simulink model "sm_motor_grader_Drive_Steer"  (R2024b)
settings: Solver=daessc  StartTime=0.0  StopTime=stopTime  RelTol=1e-3  AbsTol=1e-3  EnableMultiTasking=on
PostLoadFcn:
  | [activeTestCmds,motGradParams,stopTime] = sm_motor_grader_define_test(motGradParams,'GradingTest');
StartFcn:
  | tic
StopFcn:
  | Elapsed_Sim_Time = toc;
undefined symbols (not defined in the file): Art, LnL, LnR, motGradParams, RFL, RFR, RRL, RRR, StrL, StrR
libraries: sm_motor_grader_lib x18, sm_lib x11, nesl_utility x8, fl_lib x2, sm_vehicle_utilities_lib x2
(part 1 of 2)
settings Model: Creator=smiller  LastModifiedBy=smiller
settings SolverCC: AutoScaleAbsTol=off  MaxConsecutiveMinStep=5  AlgebraicLoopSolver=TrustRegion  MaxZcPerStep=1
settings DataIOCC: LimitDataPoints=on  MaxDataPoints=10000  ReturnWorkspaceOutputs=off  SignalLoggingName=logsout_sm_motor_grader_Drive_Steer
settings OptimizationCC: ReuseModelBlockBuffer=off  LifeSpan=inf
settings DebuggingCC: UnconnectedInputMsg=warning  UnconnectedOutputMsg=warning  UnconnectedLineMsg=warning  AllowSymbolicDim=off  SubsystemReferenceDiagnosticForUnitTest=warning  SFUnexpectedBacktrackingDiag=warning  SFNoUnconditionalDefaultTransitionDiag=warning  SFExecutionAtInitializationDiag=none  ArithmeticOperatorsInVariantConditions=warning
settings ModelReferenceCC: EnableRefExpFcnMdlSchedulingChecks=on
settings SFSimCC: SimUseLocalCustomCode=off  CustomCodeUndefinedFunction=UseInterfaceOnly
settings RTWCC: RTWUseLocalCustomCode=off  GPUComputeCapability=3.5  DLArmComputeVersion=19.05
settings CodeAppCC: StateflowObjectComments=on
settings GRTTargetCC: TargetLangStandard=C89/C90 (ANSI)
settings ConfigComp: CovMetricSettings=dw  CovSaveCumulativeToWorkspaceVar=on  CovSaveSingleToWorkspaceVar=on  CovExternalEMLEnable=off  CovSFcnEnable=off
settings SimscapeCC: SimscapeLogType=all  SimscapeLogSimulationStatistics=on  SimscapeLogName=simlog_sm_motor_grader_Drive_Steer  SimscapeLogLimitData=off  SimscapeLogDataHistory=10000
settings DiagnosticsConfigSet: SimMechanicsConflictingReferenceFrames=none
settings ExplorerConfigSet: InternalSimMechanicsExplorerSettings="<ExplorerConfiguration><canonicalview>default</canonicalview><AnimationSetting><BasePlaybackSpeed>1.0</BasePlaybackSpeed><PlaybackSpeedFactor>2.0</PlaybackSpeedFactor></AnimationSetting><TilePanel><TileInfo><Tiles Columns=\"2\" Count=\"3\" Rows=\"2\"><Column Weight=\"0.5281\"/><Column Weight=\"0.4719\"/><Row Weight=\"0.5\"/><Row Weight=\"0.5\"/><Tile Height=\"1\" Width=\"1\" X=\"0\" Y=\"0\"/><Tile Height=\"1\" Width=\"1\" X=\"0\" Y=\"1\"/><Tile Height=\"2\" Width=\"1\" X=\"1\" Y=\"0\"/></Tiles></TileInfo><SceneInfo><SceneViewer><BGColor><R>1</R><G>1</G><B>1</B></BGColor><Camera><DoPerspective>on</DoPerspective><Position><X>185.119059192113696</X><Y>-6.61432654410976184</Y><Z>13.0658786835999603</Z></Position><Center><X>185.119059192113696</X><Y>-6.61432654410976184</Y><Z>12.0658786835999603</Z></Center><Up><X>0</X><Y>1</Y><Z>0</Z></Up><ViewLimDist>1</ViewLimDist><YLim>0.466307658154998583</YLim><XLim>1.09358272855567273</XLim></Camera></SceneViewer><SceneViewer><BGColor><R>1</R><G>1</G><B>1</B></BGColor><Camera><DoPerspective>on</DoPerspective><Position><X>190.2390591921137</X><Y>-12.2143265441097615</Y><Z>2.79921201693329458</Z></Position><Center><X>189.581235564168225</X><Y>-11.4948319510444055</Y><Z>2.57651130955592267</Z></Center><Up><X>-0.15027157805512012</X><Y>0.164359538497787616</Y><Z>0.974886862632591944</Z></Up><ViewLimDist>1</ViewLimDist><YLim>0.466307658154998583</YLim><XLim>1.09358272855567273</XLim></Camera></SceneViewer><SceneViewer><BGColor><R>1</R><G>1</G><B>1</B></BGColor><Camera><DoPerspective>on</DoPerspective><Position><X>192.619059192113696</X><Y>-6.61432654410976006</Y><Z>2.66587868359996127</Z></Position><Center><X>191.641066355689389</X><Y>-6.61432654410976006</Y><Z>2.45724021182944252</Z></Center><Up><X>-0.208638471770518946</X><Y>-2.55508436632761321e-17</Y><Z>0.977992836424307566</Z></Up><ViewLimDist>1</ViewLimDist><YLim>0.466307658154998583</YLim><XLim>0.480190723283956511</XLim></Camera></SceneViewer></SceneInfo></TilePanel><MechEditorPanel><Cameras><Camera><Id>Camera1</Id><Value><Name>Track FixO FR</Name><NativeCamera><PositionTrackingFeature>Motor_Grader.Vehicle.Camera_Frames.Frame_FixO_FR.R</PositionTrackingFeature><CenterTrackingFeature>Motor_Grader.Vehicle.Camera_Frames.Frame_FixO_FR.R</CenterTrackingFeature><UpVectorTrackingFeature>Motor_Grader.Vehicle.Camera_Frames.Frame_FixO_FR.R</UpVectorTrackingFeature><CenterTrackingOrigin>off</CenterTrackingOrigin><CenterTrackingDirection>+X</CenterTrackingDirection><UpVectorTrackingDirection>+Z</UpVectorTrackingDirection></NativeCamera></Value></Camera><Camera><Id>Camera2</Id><Value><Name>Track FixO Right</Name><NativeCamera><PositionTrackingFeature>Motor_Grader.Vehicle.Camera_Frames.Frame_FixO_Right.R</PositionTrackingFeature><CenterTrackingFeature>Motor_Grader.Vehicle.Camera_Frames.Frame_FixO_Right.R</CenterTrackingFeature><UpVectorTrackingFeature>Motor_Grader.Vehicle.Camera_Frames.Frame_FixO_Right.R</UpVectorTrackingFeature><CenterTrackingOrigin>off</CenterTrackingOrigin><CenterTrackingDirection>+X</CenterTrackingDirection><UpVectorTrackingDirection>+Z</UpVectorTrackingDirection></NativeCamera></Value></Camera><Camera><Id>Camera3</Id><Value><Name>Track FixO RR</Name><NativeCamera><PositionTrackingFeature>Motor_Grader.Vehicle.Camera_Frames.Frame_FixO_RR.R</PositionTrackingFeature><CenterTrackingFeature>Motor_Grader.Vehicle.Camera_Frames.Frame_FixO_RR.R</CenterTrackingFeature><UpVectorTrackingFeature>Motor_Grader.Vehicle.Camera_Frames.Frame_FixO_RR.R</UpVectorTrackingFeature><CenterTrackingOrigin>off</CenterTrackingOrigin><CenterTrackingDirection>+X</CenterTrackingDirection><UpVectorTrackingDirection>+Z</UpVectorTrackingDirection></NativeCamera></Value></Camera><Camera><Id>Camera4</Id><Value><Name>Track FixO RL</Name><NativeCamera><PositionTrackingFeature>Motor_Grader.Vehicle.Camera_Frames.Frame_FixO_RL.R</PositionTrackingFeature><CenterTrackingFeature>Motor_Grader.Vehicle.Camera_Frames.Frame_FixO_RL.R</CenterTrackingFeature><UpVectorTrackingFeature>Motor_Grader.Vehicle.Camera_Frames.Frame_FixO_RL.R</UpVectorTrackingFeature><CenterTrackingOrigin>off</CenterTrackingOrigin><CenterTrackingDirection>+X</CenterTrackingDirection><UpVectorTrackingDirection>+Z</UpVectorTrackingDirection></NativeCamera></Value></Camera><Camera><Id>Camera5</Id><Value><Name>Track FixO Left</Name><NativeCamera><PositionTrackingFeature>Motor_Grader.Vehicle.Camera_Frames.Frame_FixO_Left.R</PositionTrackingFeature><CenterTrackingFeature>Motor_Grader.Vehicle.Camera_Frames.Frame_FixO_Left.R</CenterTrackingFeature><UpVectorTrackingFeature>Motor_Grader.Vehicle.Camera_Frames.Frame_FixO_Left.R</UpVectorTrackingFeature><CenterTrackingOrigin>off</CenterTrackingOrigin><CenterTrackingDirection>+X</CenterTrackingDirection><UpVectorTrackingDirection>+Z</UpVectorTrackingDirection></NativeCamera></Value></Camera><Camera><Id>Camera6</Id><Value><Name>Track FixO FL</Name><NativeCamera><PositionTrackingFeature>Motor_Grader.Vehicle.Camera_Frames.Frame_FixO_FL.R</PositionTrackingFeature><CenterTrackingFeature>Motor_Grader.Vehicle.Camera_Frames.Frame_FixO_FL.R</CenterTrackingFeature><UpVectorTrackingFeature>Motor_Grader.Vehicle.Camera_Frames.Frame_FixO_FL.R</UpVectorTrackingFeature><CenterTrackingOrigin>off</CenterTrackingOrigin><CenterTrackingDirection>+X</CenterTrackingDirection><UpVectorTrackingDirection>+Z</UpVectorTrackingDirection></NativeCamera></Value></Camera><Camera><Id>Camera7</Id><Value><Name>Track FixO Top</Name><NativeCamera><PositionTrackingFeature>Motor_Grader.Vehicle.Camera_Frames.Frame_FixO_Top.R</PositionTrackingFeature><CenterTrackingFeature>Motor_Grader.Vehicle.Camera_Frames.Frame_FixO_Top.R</CenterTrackingFeature><UpVectorTrackingFeature>Motor_Grader.Vehicle.Camera_Frames.Frame_FixO_Top.R</UpVectorTrackingFeature><CenterTrackingOrigin>off</CenterTrackingOrigin><CenterTrackingDirection>+X</CenterTrackingDirection><UpVectorTrackingDirection>+Z</UpVectorTrackingDirection></NativeCamera></Value></Camera><Camera><Id>Camera8</Id><Value><Name>Track FixO Front</Name><NativeCamera><PositionTrackingFeature>Motor_Grader.Vehicle.Camera_Frames.Frame_FixO_Front.R</PositionTrackingFeature><CenterTrackingFeature>Motor_Grader.Vehicle.Camera_Frames.Frame_FixO_Front.R</CenterTrackingFeature><UpVectorTrackingFeature>Motor_Grader.Vehicle.Camera_Frames.Frame_FixO_Front.R</UpVectorTrackingFeature><CenterTrackingOrigin>off</CenterTrackingOrigin><CenterTrackingDirection>+X</CenterTrackingDirection><UpVectorTrackingDirection>+Z</UpVectorTrackingDirection></NativeCamera></Value></Camera><Camera><Id>Camera9</Id><Value><Name>Track FixO Rear</Name><NativeCamera><PositionTrackingFeature>Motor_Grader.Vehicle.Camera_Frames.Frame_FixO_Rear.R</PositionTrackingFeature><CenterTrackingFeature>Motor_Grader.Vehicle.Camera_Frames.Frame_FixO_Rear.R</CenterTrackingFeature><UpVectorTrackingFeature>Motor_Grader.Vehicle.Camera_Frames.Frame_FixO_Rear.R</UpVectorTrackingFeature><CenterTrackingOrigin>off</CenterTrackingOrigin><CenterTrackingDirection>+X</CenterTrackingDirection><UpVectorTrackingDirection>+Z</UpVectorTrackingDirection></NativeCamera></Value></Camera><Camera><Id>Camera10</Id><Value><Name>Track FR</Name><NativeCamera><PositionTrackingFeature>Motor_Grader.Vehicle.Camera_Frames.Frame_FR.R</PositionTrackingFeature><CenterTrackingFeature>Motor_Grader.Vehicle.Camera_Frames.Frame_FR.R</CenterTrackingFeature><UpVectorTrackingFeature>Motor_Grader.Vehicle.Camera_Frames.Frame_FR.R</UpVectorTrackingFeature><CenterTrackingOrigin>off</CenterTrackingOrigin><CenterTrackingDirection>+X</CenterTrackingDirection><UpVectorTrackingDirection>+Z</UpVectorTrackingDirection></NativeCamera></Value></Camera><Camera><Id>Camera11</Id><Value><Name>Track Right</Name><NativeCamera><PositionTrackingFeature>Motor_Grader.Vehicle.Camera_Frames.Frame_Right.R</PositionTrackingFeature><CenterTrackingFeature>Motor_Grader.Vehicle.Camera_Frames.Frame_Right.R</CenterTrackingFeature><UpVectorTrackingFeature>Motor_Grader.Vehicle.Camera_Frames.Frame_Right.R</UpVectorTrackingFeature><CenterTrackingOrigin>off</CenterTrackingOrigin><CenterTrackingDirection>+X</CenterTrackingDirection><UpVectorTrackingDirection>+Z</UpVectorTrackingDirection></NativeCamera></Value></Camera><Camera><Id>Camera12</Id><Value><Name>Track RR</Name><NativeCamera><PositionTrackingFeature>Motor_Grader.Vehicle.Camera_Frames.Frame_RR.R</PositionTrackingFeature><CenterTrackingFeature>Motor_Grader.Vehicle.Camera_Frames.Frame_RR.R</CenterTrackingFeature><UpVectorTrackingFeature>Motor_Grader.Vehicle.Camera_Frames.Frame_RR.R</UpVectorTrackingFeature><CenterTrackingOrigin>off</CenterTrackingOrigin><CenterTrackingDirection>+X</CenterTrackingDirection><UpVectorTrackingDirection>+Z</UpVectorTrackingDirection></NativeCamera></Value></Camera><Camera><Id>Camera13</Id><Value><Name>Track RL</Name><NativeCamera><PositionTrackingFeature>Motor_Grader.Vehicle.Camera_Frames.Frame_RL.R</PositionTrackingFeature><CenterTrackingFeature>Motor_Grader.Vehicle.Camera_Frames.Frame_RL.R</CenterTrackingFeature><UpVectorTrackingFeature>Motor_Grader.Vehicle.Camera_Frames.Frame_RL.R</UpVectorTrackingFeature><CenterTrackingOrigin>off</CenterTrackingOrigin><CenterTrackingDirection>+X</CenterTrackingDirection><UpVectorTrackingDirection>+Z</UpVectorTrackingDirection></NativeCamera></Value></Camera><Camera><Id>Camera14</Id><Value><Name>Track Left</Name><NativeCamera><PositionTrackingFeature>Motor_Grader.Vehicle.Camera_Frames.Frame_Left.R</PositionTrackingFeature><CenterTrackingFeature>Motor_Grader.Vehicle.Camera_Frames.Frame_Left.R</CenterTrackingFeature><UpVectorTrackingFeature>Motor_Grader.Vehicle.Camera_Frames.Frame_Left.R</UpVectorTrackingFeature><CenterTrackingOrigin>off</CenterTrackingOrigin><CenterTrackingDirection>+X</CenterTrackingDirection><UpVectorTrackingDirection>+Z</UpVectorTrackingDirection></NativeCamera></Value></Camera><Camera><Id>Camera15</Id><Value><Name>Track FL</Name><NativeCamera><PositionTrackingFeature>Motor_Grader.Vehicle.Camera_Frames.Frame_FL.R</PositionTrackingFeature><CenterTrackingFeature>Motor_Grader.Vehicle.Camera_Frames.Frame_FL.R</CenterTrackingFeature><UpVectorTrackingFeature>Motor_Grader.Vehicle.Camera_Frames.Frame_FL.R</UpVectorTrackingFeature><CenterTrackingOrigin>off</CenterTrackingOrigin><CenterTrackingDirection>+X</CenterTrackingDirection><UpVectorTrackingDirection>+Z</UpVectorTrackingDirection></NativeCamera></Value></Camera><Camera><Id>Camera16</Id><Value><Name>Track Top</Name><NativeCamera><PositionTrackingFeature>Motor_Grader.Vehicle.Camera_Frames.Frame_Top.R</PositionTrackingFeature><CenterTrackingFeature>Motor_Grader.Vehicle.Camera_Frames.Frame_Top.R</CenterTrackingFeature><UpVectorTrackingFeature>Motor_Grader.Vehicle.Camera_Frames.Frame_Top.R</UpVectorTrackingFeature><CenterTrackingOrigin>off</CenterTrackingOrigin><CenterTrackingDirection>+X</CenterTrackingDirection><UpVectorTrackingDirection>+Z</UpVectorTrackingDirection></NativeCamera></Value></Camera><Camera><Id>Camera17</Id><Value><Name>Track Front</Name><NativeCamera><PositionTrackingFeature>Motor_Grader.Vehicle.Camera_Frames.Frame_Front.R</PositionTrackingFeature><CenterTrackingFeature>Motor_Grader.Vehicle.Camera_Frames.Frame_Front.R</CenterTrackingFeature><UpVectorTrackingFeature>Motor_Grader.Vehicle.Camera_Frames.Frame_Front.R</UpVectorTrackingFeature><CenterTrackingOrigin>off</CenterTrackingOrigin><CenterTrackingDirection>+X</CenterTrackingDirection><UpVectorTrackingDirection>+Z</UpVectorTrackingDirection></NativeCamera></Value></Camera><Camera><Id>Camera18</Id><Value><Name>Track Rear</Name><NativeCamera><PositionTrackingFeature>Motor_Grader.Vehicle.Camera_Frames.Frame_Rear.R</PositionTrackingFeature><CenterTrackingFeature>Motor_Grader.Vehicle.Camera_Frames.Frame_Rear.R</CenterTrackingFeature><UpVectorTrackingFeature>Motor_Grader.Vehicle.Camera_Frames.Frame_Rear.R</UpVectorTrackingFeature><CenterTrackingOrigin>off</CenterTrackingOrigin><CenterTrackingDirection>+X</CenterTrackingDirection><UpVectorTrackingDirection>+Z</UpVectorTrackingDirection></NativeCamera></Value></Camera><Camera><Id>Camera19</Id><Value><Name>Track Blade Front</Name><NativeCamera><PositionTrackingFeature>Motor_Grader.Vehicle.Camera_Frames.Frame_SuspF.R</PositionTrackingFeature><CenterTrackingFeature>Motor_Grader.Vehicle.Camera_Frames.Frame_SuspF.R</CenterTrackingFeature><UpVectorTrackingFeature>Motor_Grader.Vehicle.Camera_Frames.Frame_SuspF.R</UpVectorTrackingFeature><CenterTrackingOrigin>off</CenterTrackingOrigin><CenterTrackingDirection>+X</CenterTrackingDirection><UpVectorTrackingDirection>+Z</UpVectorTrackingDirection></NativeCamera></Value></Camera><Camera><Id>Camera20</Id><Value><Name>Track Blade Rear</Name><NativeCamera><PositionTrackingFeature>Motor_Grader.Vehicle.Camera_Frames.Frame_SuspR.R</PositionTrackingFeature><CenterTrackingFeature>Motor_Grader.Vehicle.Camera_Frames.Frame_SuspR.R</CenterTrackingFeature><UpVectorTrackingFeature>Motor_Grader.Vehicle.Camera_Frames.Frame_SuspR.R</UpVectorTrackingFeature><CenterTrackingOrigin>off</CenterTrackingOrigin><CenterTrackingDirection>+X</CenterTrackingDirection><UpVectorTrackingDirection>+Z</UpVectorTrackingDirection></NativeCamera></Value></Camera><Camera><Id>Camera21</Id><Value><Name>Track Wheel FR</Name><NativeCamera><PositionTrackingFeature>Motor_Grader.Vehicle.Camera_Frames.Frame_Wheel_FR.R</PositionTrackingFeature><CenterTrackingFeature>Motor_Grader.Vehicle.Camera_Frames.Frame_Wheel_FR.R</CenterTrackingFeature><UpVectorTrackingFeature>Motor_Grader.Vehicle.Camera_Frames.Frame_Wheel_FR.R</UpVectorTrackingFeature><CenterTrackingOrigin>off</CenterTrackingOrigin><CenterTrackingDirection>+X</CenterTrackingDirection><UpVectorTrackingDirection>+Z</UpVectorTrackingDirection></NativeCamera></Value></Camera><Camera><Id>Camera22</Id><Value><Name>Track Blade Right</Name><NativeCamera><PositionTrackingFeature>Motor_Grader.Vehicle.Camera_Frames.Frame_Wheel_RR.R</PositionTrackingFeature><CenterTrackingFeature>Motor_Grader.Vehicle.Camera_Frames.Frame_Wheel_RR.R</CenterTrackingFeature><UpVectorTrackingFeature>Motor_Grader.Vehicle.Camera_Frames.Frame_Wheel_RR.R</UpVectorTrackingFeature><CenterTrackingOrigin>off</CenterTrackingOrigin><CenterTrackingDirection>+X</CenterTrackingDirection><UpVectorTrackingDirection>+Z</UpVectorTrackingDirection></NativeCamera></Value></Camera><Camera><Id>Camera23</Id><Value><Name>Track Blade Left</Name><NativeCamera><PositionTrackingFeature>Motor_Grader.Vehicle.Camera_Frames.Frame_Wheel_RL.R</PositionTrackingFeature><CenterTrackingFeature>Motor_Grader.Vehicle.Camera_Frames.Frame_Wheel_RL.R</CenterTrackingFeature><UpVectorTrackingFeature>Motor_Grader.Vehicle.Camera_Frames.Frame_Wheel_RL.R</UpVectorTrackingFeature><CenterTrackingOrigin>off</CenterTrackingOrigin><CenterTrackingDirection>+X</CenterTrackingDirection><UpVectorTrackingDirection>+Z</UpVectorTrackingDirection></NativeCamera></Value></Camera><Camera><Id>Camera24</Id><Value><Name>Track Wheel FL</Name><NativeCamera><PositionTrackingFeature>Motor_Grader.Vehicle.Camera_Frames.Frame_Wheel_FL.R</PositionTrackingFeature><CenterTrackingFeature>Motor_Grader.Vehicle.Camera_Frames.Frame_Wheel_FL.R</CenterTrackingFeature><UpVectorTrackingFeature>Motor_Grader.Vehicle.Camera_Frames.Frame_Wheel_FL.R</UpVectorTrackingFeature><CenterTrackingOrigin>off</CenterTrackingOrigin><CenterTrackingDirection>+X</CenterTrackingDirection><UpVectorTrackingDirection>+Z</UpVectorTrackingDirection></NativeCamera></Value></Camera><Camera><Id>Camera25</Id><Value><Name>View Seat</Name><NativeCamera><PositionTrackingFeature>Motor_Grader.Vehicle.Camera_Frames.Frame_View_Seat_FL.R</PositionTrackingFeature><CenterTrackingFeature>Motor_Grader.Vehicle.Camera_Frames.Frame_View_Seat_FL.R</CenterTrackingFeature><UpVectorTrackingFeature>Motor_Grader.Vehicle.Camera_Frames.Frame_View_Seat_FL.R</UpVectorTrackingFeature><CenterTrackingOrigin>off</CenterTrackingOrigin><CenterTrackingDirection>+X</CenterTrackingDirection><UpVectorTrackingDirection>+Z</UpVectorTrackingDirection></NativeCamera></Value></Camera><Camera><Id>Camera26</Id><Value><Name>View Seat FR</Name><NativeCamera><PositionTrackingFeature>Motor_Grader.Vehicle.Camera_Frames.Frame_View_Seat_FR.R</PositionTrackingFeature><CenterTrackingFeature>Motor_Grader.Vehicle.Camera_Frames.Frame_View_Seat_FR.R</CenterTrackingFeature><UpVectorTrackingFeature>Motor_Grader.Vehicle.Camera_Frames.Frame_View_Seat_FR.R</UpVectorTrackingFeature><CenterTrackingOrigin>off</CenterTrackingOrigin><CenterTrackingDirection>+X</CenterTrackingDirection><UpVectorTrackingDirection>+Z</UpVectorTrackingDirection></NativeCamera></Value></Camera><Camera><Id>Camera27</Id><Value><Name>View Susp FR</Name><NativeCamera><PositionTrackingFeature>Motor_Grader.Vehicle.Camera_Frames.Frame_View_Susp_FR.R</PositionTrackingFeature><CenterTrackingFeature>Motor_Grader.Vehicle.Camera_Frames.Frame_View_Susp_FR.R</CenterTrackingFeature><UpVectorTrackingFeature>Motor_Grader.Vehicle.Camera_Frames.Frame_View_Susp_FR.R</UpVectorTrackingFeature><CenterTrackingOrigin>off</CenterTrackingOrigin><CenterTrackingDirection>+X</CenterTrackingDirection><UpVectorTrackingDirection>+Z</UpVectorTrackingDirection></NativeCamera></Value></Camera><Camera><Id>Camera28</Id><Value><Name>View SaddleR</Name><NativeCamera><PositionTrackingFeature>Motor_Grader.Vehicle.Camera_Frames.Frame_View_Susp_RR.R</PositionTrackingFeature><CenterTrackingFeature>Motor_Grader.Vehicle.Camera_Frames.Frame_View_Susp_RR.R</CenterTrackingFeature><UpVectorTrackingFeature>Motor_Grader.Vehicle.Camera_Frames.Frame_View_Susp_RR.R</UpVectorTrackingFeature><CenterTrackingOrigin>off</CenterTrackingOrigin><CenterTrackingDirection>+X</CenterTrackingDirection><UpVectorTrackingDirection>+Z</UpVectorTrackingDirection></NativeCamera></Value></Camera><Camera><Id>Camera29</Id><Value><Name>View SaddleL</Name><NativeCamera><PositionTrackingFeature>Motor_Grader.Vehicle.Camera_Frames.Frame_View_Susp_RL.R</PositionTrackingFeature><CenterTrackingFeature>Motor_Grader.Vehicle.Camera_Frames.Frame_View_Susp_RL.R</CenterTrackingFeature><UpVectorTrackingFeature>Motor_Grader.Vehicle.Camera_Frames.Frame_View_Susp_RL.R</UpVectorTrackingFeature><CenterTrackingOrigin>off</CenterTrackingOrigin><CenterTrackingDirection>+X</CenterTrackingDirection><UpVectorTrackingDirection>+Z</UpVectorTrackingDirection></NativeCamera></Value></Camera><Camera><Id>Camera30</Id><Value><Name>View Susp FL</Name><NativeCamera><PositionTrackingFeature>Motor_Grader.Vehicle.Camera_Frames.Frame_View_Susp_FL.R</PositionTrackingFeature><CenterTrackingFeature>Motor_Grader.Vehicle.Camera_Frames.Frame_View_Susp_FL.R</CenterTrackingFeature><UpVectorTrackingFeature>Motor_Grader.Vehicle.Camera_Frames.Frame_View_Susp_FL.R</UpVectorTrackingFeature><CenterTrackingOrigin>off</CenterTrackingOrigin><CenterTrackingDirection>+X</CenterTrackingDirection><UpVectorTrackingDirection>+Z</UpVectorTrackingDirection></NativeCamera></Value></Camera><Camera><Id>Camera31</Id><Value><Name>Dolly Camera</Name><NativeCamera><PositionTrackingFeature>Motor_Grader.Vehicle.Camera_Frames.Frame_Dolly.R</PositionTrackingFeature><CenterTrackingFeature>Motor_Grader.Vehicle.Camera_Frames.Frame_Dolly.R</CenterTrackingFeature><UpVectorTrackingFeature>Motor_Grader.Vehicle.Camera_Frames.Frame_Dolly.R</UpVectorTrackingFeature><CenterTrackingOrigin>off</CenterTrackingOrigin><CenterTrackingDirection>+X</CenterTrackingDirection><UpVectorTrackingDirection>+Z</UpVectorTrackingDirection></NativeCamera></Value></Camera><Camera><Id>Camera32</Id><Value><Name>Track Dolly Camera</Name><NativeCamera><PositionTrackingFeature>Motor_Grader.Vehicle.Camera_Frames.Frame_Dolly.R</PositionTrackingFeature><CenterTrackingFeature>Motor_Grader.Vehicle.Camera_Frames.Transform_Camera_Ref.F</CenterTrackingFeature><UpVectorTrackingFeature>Motor_Grader.Vehicle.Camera_Frames.World_Frame.W</UpVectorTrackingFeature><CenterTrackingOrigin>on</CenterTrackingOrigin><UpVectorTrackingDirection>+Z</UpVectorTrackingDirection></NativeCamera></Value></Camera></Cameras><GfxPanelCameraMap><MapElement CameraMLId=\"Camera7\" GfxPanelIndex=\"0\"/><MapElement CameraMLId=\"Camera1\" GfxPanelIndex=\"1\"/><MapElement CameraMLId=\"Camera8\" GfxPanelIndex=\"2\"/></GfxPanelCameraMap><VideoCreator><PlaybackSpeedRatio>1.0</PlaybackSpeedRatio><FrameRate>30</FrameRate><VideoFormat>MPEG-4</VideoFormat><FrameSize>[800 450]</FrameSize></VideoCreator></MechEditorPanel></ExplorerConfiguration>"

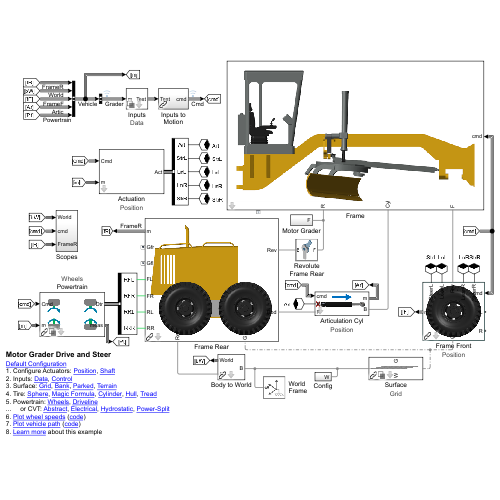
[thumbnail: Simulink's stored preview of the top-level diagram]
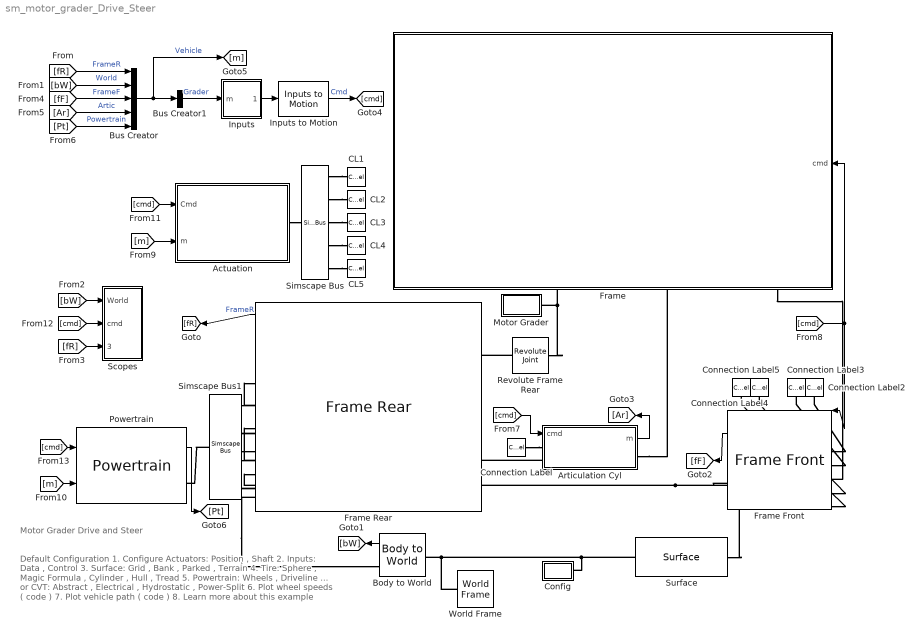
== system sm_motor_grader_Drive_Steer ==
  note: Motor Grader Drive and Steer
  note: Default Configuration
      | 1. Configure Actuators: Position , Shaft
      | 2. Inputs: Data , Control
      | 3. Surface: Grid , Bank , Parked , Terrain
      | 4. Tire: Sphere , Magic Formula , Cylinder , Hull , Tread
      | 5. Powertrain: Wheels , Driveline
      | ... or CVT: Abstract , Electrical , Hydrostatic , Power-Split
      | 6. Plot wheel speeds ( code )
      | 7. Plot vehicle path ( code )
      | 8. Learn more about this example
  Actuation : Subsystem  VariantControl=Actuation  mask{popup_actuator_model=Position}
      mask prompts: popup_actuator_model "Actuation Mode"
      mask init:
      | bh = gcb;
      | modestr = get_param(bh,'popup_actuator_model');
      | 
      | set_param([bh '/Actuator SteerL'],'LabelModeActiveChoice',modestr)
      | set_param([bh '/Actuator SteerR'],'LabelModeActiveChoice',modestr)
      | set_param([bh '/Actuator LeanL'],'LabelModeActiveChoice',modestr)
      | set_param([bh '/Actuator LeanR'],'LabelModeActiveChoice',modestr)
      settings: AttributesFormatString=%<popup_actuator_model>
      mask TypeOptions popup_actuator_model: Position | Shaft
  Articulation Cyl : Subsystem  mask{popup_actuator_model=Position}
      mask prompts: popup_actuator_model "Actuation Mode"
      mask init:
      | bh = gcb;
      | if(strcmp(get_param(bh,'popup_actuator_model'),'Shaft'))
      |     set_param([bh '/Actuator'],'LabelModeActiveChoice','Shaft')
      | else
      |     set_param([bh '/Actuator'],'LabelModeActiveChoice','Position')
      | end
      settings: AttributesFormatString=%<popup_actuator_model>
      mask TypeOptions popup_actuator_model: Position | Shaft
      mask Display:
      | bh = gcb;
      | if(strcmp(get_param(bh,'popup_actuator_model'),'Position'))
      |     image('sm_motor_grader_actuator_intfPosition_IMAGE.png')
      | else
      |     image('sm_motor_grader_actuator_intfShaft_IMAGE.png')
      | end
      | %image('sm_motor_grader_articCylRod_IMAGE.png')
  Body to World : sm_vehicle_utilities_lib/Body to World  Init=Init.Vehicle  SpecifyPosTarget=on
  Bus Creator : BusCreator  Inputs=5
  Bus Creator1 : BusCreator  Inputs=1
  CL1 : ConnectionLabel  Label=Art
  CL2 : ConnectionLabel  Label=StrL
  CL3 : ConnectionLabel  Label=LnL
  CL4 : ConnectionLabel  Label=LnR
  CL5 : ConnectionLabel  Label=StrR
  Config : Subsystem
  Connection Label : ConnectionLabel  Label=Art
  Connection Label2 : ConnectionLabel  Label=StrR
  Connection Label3 : ConnectionLabel  Label=LnR
  Connection Label4 : ConnectionLabel  Label=LnL
  Connection Label5 : ConnectionLabel  Label=StrL
  Frame : Subsystem
      settings: PortSchema="{\"entries\":[{\"content\":{\"sides\":[{\"content\":{},\"type\":\"ConnectorPlacement.EquallySpacedRectSide\",\"uuid\":\"956ff1aa-cf24-496e-9779-d98cb55dab7e\"},{\"content\":{\"connectorIds\":[\"RConn1\",\"RConn2\",\"RConn3\",\"RConn4\"],\"side\":\"RIGHT\"},\"type\":\"ConnectorPlacement.EquallySpacedRectSide\",\"uuid\":\"9c9b4268-8eee-41b9-b50a-4033054aa2f0\"},{\"content\":{\"side\":\"TOP\"},\"type\":\"ConnectorPlacement.EquallySpacedRectSide\",\"uuid\":\"ed4b7b74-ed0a-49ca-b139-bba335fa3413\"},{\"content\":{\"connectorIds\":[\"In1\"],\"side\":\"BOTTOM\"},\"type\":\"ConnectorPlacement.EquallySpacedRectSide\",\"uuid\":\"cd037d6e-8d6c-4a0e-a629-b4586db15f4a\"}]},\"type\":\"ConnectorPlacement.EquallySpacedConnector\",\"uuid\":\"3490148e-7dca-48b7-9597-0781f6c140f1\"}],\"packageUris\":[\"http://schema.mathworks.com/mf0/Connector/R2020b\"],\"version\":\"1.0\"}"
      mask Display: image('sm_motor_grader_frameCabBlade_IMAGE.png')
  Frame Front : sm_motor_grader_lib/Frame Front  popup_actuator_model=Position  popup_ground_contact=Magic Formula
      settings: AttributesFormatString=%<popup_actuator_model>
  Frame Rear : sm_motor_grader_lib/Frame Rear  popup_ground_contact=Magic Formula
  Inputs : Subsystem  Variant=on  VariantControlMode=label  VariantControl=Inputs  LabelModeActiveChoice=Data  mask{test_source=Data}
      mask prompts: test_source "Test Source"
      mask init:
      | bh = gcb;
      | data_source = get_param(bh,'test_source');
      | set_param(bh,'LabelModeActiveChoice',data_source)
      settings: AttributesFormatString=%<LabelModeActiveChoice>
      mask TypeOptions test_source: Data | Control
      mask Display: disp(' ')
  Inputs to Motion : sm_motor_grader_lib/Inputs to Motion  SystemSampleTime=-1  VariantActivationTime=update diagram  AllowFlexibleInterface=on  Latency=0  AutoFrameSizeCalculation=off
  Motor Grader : Subsystem
  Powertrain : sm_motor_grader_lib/Powertrain  VariantControl=Powertrain  LabelModeActiveChoice=Torque4  popup_powertrain_config=Wheels
      settings: AttributesFormatString=%<popup_powertrain_config>
  Revolute Frame Rear : sm_lib/Joints/Revolute Joint  JointMode=Normal  CompositeWrenchDir=FollowerOnBase  CompositeWrenchFrame=BaseFrame  SenseConstraintForce=off  SenseConstraintTorque=off  SenseTotalForce=off  SenseTotalTorque=off  PositionTargetSpecify=on  PositionTargetPriority=Low  PositionTargetValue=0  PositionTargetValueUnits=deg  VelocityTargetSpecify=off  VelocityTargetPriority=High  VelocityTargetValue=0  VelocityTargetValueUnits=deg/s  EquilibriumPosition=0  EquilibriumPositionUnits=deg  SpringStiffness=0  SpringStiffnessUnits=N*m/deg  DampingCoefficient=0  DampingCoefficientUnits=N*m/(deg/s)  LowerLimitSpecify=off  LowerLimitBound=-90  LowerLimitBoundUnits=deg  LowerLimitStiffness=1e4  LowerLimitStiffnessUnits=N*m/deg  LowerLimitDamping=10  LowerLimitDampingUnits=N*m/(deg/s)  LowerLimitTransitionRegionWidth=0.1  LowerLimitTransitionRegionWidthUnits=deg  UpperLimitSpecify=off  UpperLimitBound=90  UpperLimitBoundUnits=deg  UpperLimitStiffness=1e4  UpperLimitStiffnessUnits=N*m/deg  UpperLimitDamping=10  UpperLimitDampingUnits=N*m/(deg/s)  UpperLimitTransitionRegionWidth=0.1  UpperLimitTransitionRegionWidthUnits=deg  TorqueActuationMode=NoTorque  MotionActuationMode=ComputedMotion  SensePosition=off  SenseVelocity=off  SenseAcceleration=off  SenseTorqueForce=off  SenseLowerLimitTorqueForce=off  SenseUpperLimitTorqueForce=off
  Scopes : Subsystem
  Simscape Bus : SimscapeBus  HierarchyStrings=Art;StrL;LnL;LnR;StrR
  Simscape Bus1 : SimscapeBus  HierarchyStrings=RFL;RFR;RRL;RRR
  Surface : sm_motor_grader_lib/Surface  VariantControl=Grid  LabelModeActiveChoice=Grid  popup_surface_type=Grid
      settings: AttributesFormatString=%<popup_surface_type>
  World Frame : sm_lib/Frames and Transforms/World Frame
  wires:
  Frame Rear/1 -> [fR]  "FrameR"
  Bus Creator1/1 -> Inputs/1(m)  "Grader"
  Inputs to Motion/1 -> [cmd]  "Cmd"
  [fR] -> Bus Creator/1  "FrameR"
  Body to World/1 -> [bW]
  [bW] -> Bus Creator/2  "World"
  Articulation Cyl/1(m) -> [Ar]
  Frame Front/1 -> [fF]
  Inputs/1(Test) -> Inputs to Motion/1
  [fF] -> Bus Creator/3  "FrameF"
  [Ar] -> Bus Creator/4  "Artic"
  [cmd] -> Frame Front/1, Frame/1(cmd)
  [cmd] -> Articulation Cyl/1(cmd)
  [m] -> Actuation/2(m)
  [m] -> Powertrain/2
  [cmd] -> Actuation/1(Cmd)
  [cmd] -> Powertrain/1
  [bW] -> Scopes/1(World)
  [cmd] -> Scopes/2(cmd)
  [fR] -> Scopes/3(FrameR)
  Bus Creator/1 -> [m], Bus Creator1/1  "Vehicle"
  Powertrain/1 -> [Pt]
  [Pt] -> Bus Creator/5  "Powertrain"
  connections:
  Simscape Bus1/RConn1 -- Powertrain/RConn1
  Revolute Frame Rear/LConn1 -- Frame Rear/LConn1
  World Frame/RConn1 -- Surface/LConn1 -- Config/LConn1 -- Body to World/LConn1
  Frame Rear/RConn8 -- Body to World/RConn1
  Frame Front/RConn1 -- Surface/RConn1 -- Frame Rear/RConn7
  Frame Front/LConn6 -- Connection Label4/LConn1
  Frame Front/LConn3 -- Connection Label2/LConn1
  Frame Front/LConn7 -- Connection Label5/LConn1
  Frame Front/LConn4 -- Connection Label3/LConn1
  Revolute Frame Rear/RConn1 -- Frame/RConn2 -- Motor Grader/RConn1
  Articulation Cyl/LConn2 -- Frame Rear/LConn2
  Articulation Cyl/RConn1 -- Frame/RConn3
  Simscape Bus1/LConn1 -- Frame Rear/RConn3
  Simscape Bus1/LConn2 -- Frame Rear/RConn4
  Simscape Bus1/LConn3 -- Frame Rear/RConn5
  Simscape Bus1/LConn4 -- Frame Rear/RConn6
  Actuation/RConn1 -- Simscape Bus/RConn1
  Simscape Bus/LConn4 -- CL4/LConn1
  Simscape Bus/LConn5 -- CL5/LConn1
  Simscape Bus/LConn2 -- CL2/LConn1
  Simscape Bus/LConn1 -- CL1/LConn1
  Simscape Bus/LConn3 -- CL3/LConn1
  Connection Label/LConn1 -- Articulation Cyl/LConn1
  Frame/RConn4 -- Frame Front/LConn5

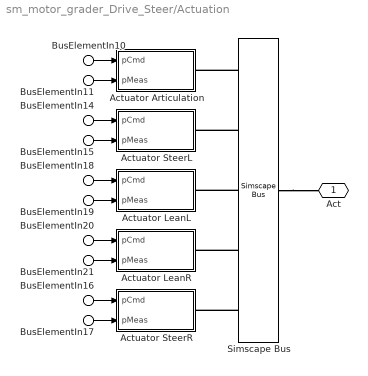
== system sm_motor_grader_Drive_Steer/Actuation ==
  BusElementIn10 : Inport  PortName=Cmd  Element=pArtic
  BusElementIn14 : Inport  PortName=Cmd  Element=pSteerL
  BusElementIn16 : Inport  PortName=Cmd  Element=pSteerR
  BusElementIn18 : Inport  PortName=Cmd  Element=pLeanL
  BusElementIn20 : Inport  PortName=Cmd  Element=pLeanR
  BusElementIn11 : Inport  Port=2  PortName=m  Element=Artic.p
  BusElementIn15 : Inport  Port=2  PortName=m  Element=FrameF.SteerL.p
  BusElementIn19 : Inport  Port=2  PortName=m  Element=FrameF.LeanL.p
  BusElementIn21 : Inport  Port=2  PortName=m  Element=FrameF.LeanR.p
  BusElementIn17 : Inport  Port=2  PortName=m  Element=FrameF.SteerR.p
  Actuator Articulation : Subsystem  Variant=on  VariantControlMode=label  VariantControl=Actuator Articulation  LabelModeActiveChoice=Position
  Actuator LeanL : Subsystem  Variant=on  VariantControlMode=label  VariantControl=Actuator LeanL  LabelModeActiveChoice=Position
  Actuator LeanR : Subsystem  Variant=on  VariantControlMode=label  VariantControl=Actuator LeanR  LabelModeActiveChoice=Position
  Actuator SteerL : Subsystem  Variant=on  VariantControlMode=label  VariantControl=Actuator SteerL  LabelModeActiveChoice=Position
  Actuator SteerR : Subsystem  Variant=on  VariantControlMode=label  VariantControl=Actuator SteerR  LabelModeActiveChoice=Position
  Simscape Bus : SimscapeBus  HierarchyStrings=Art;StrL;LnL;LnR;StrR
  Act : PMIOPort  Side=Right
  wires:
  BusElementIn21/1 -> Actuator LeanR/2(pMeas)
  BusElementIn20/1 -> Actuator LeanR/1(pCmd)
  BusElementIn19/1 -> Actuator LeanL/2(pMeas)
  BusElementIn18/1 -> Actuator LeanL/1(pCmd)
  BusElementIn17/1 -> Actuator SteerR/2(pMeas)
  BusElementIn16/1 -> Actuator SteerR/1(pCmd)
  BusElementIn15/1 -> Actuator SteerL/2(pMeas)
  BusElementIn14/1 -> Actuator SteerL/1(pCmd)
  BusElementIn11/1 -> Actuator Articulation/2(pMeas)
  BusElementIn10/1 -> Actuator Articulation/1(pCmd)
  connections:
  Simscape Bus/LConn4 -- Actuator LeanR/RConn1
  Simscape Bus/LConn3 -- Actuator LeanL/RConn1
  Simscape Bus/LConn5 -- Actuator SteerR/RConn1
  Simscape Bus/LConn2 -- Actuator SteerL/RConn1
  Simscape Bus/LConn1 -- Actuator Articulation/RConn1
  Simscape Bus/RConn1 -- Act/RConn1

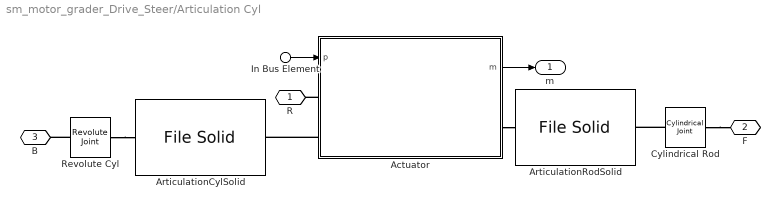
== system sm_motor_grader_Drive_Steer/Articulation Cyl ==
  In Bus Element : Inport  PortName=cmd  Element=pArtic
  Actuator : Subsystem  Variant=on  VariantControlMode=label  VariantControl=Position  LabelModeActiveChoice=Position
  ArticulationCylSolid : sm_lib/Body Elements/File Solid  ExtGeomFileName=ArticulationCylinder.step  UnitType=FromFile  ExtGeomFileUnits=m  StepReaderType=HEX  ExportConvexHullGeometry=off  InertiaType=CalculateFromGeometry  BasedOnType=Mass  Density=1000  DensityUnits=kg/m^3  Mass=motGradParams.articulation.cyl.mass  MassUnits=kg  CenterOfMass=[0 0 0]  CenterOfMassUnits=m  MomentsOfInertia=[1 1 1]  MomentsOfInertiaUnits=kg*m^2  ProductsOfInertia=[0 0 0]  ProductsOfInertiaUnits=kg*m^2  GraphicType=FromGeometry  MarkerShape=Sphere  MarkerSize=10  GraphicVisPropType=SimpleVisualProperties  GraphicDiffuseColor=mtrgrd.clr.artic_cyl  GraphicOpacity=0.5  GraphicSpecularColor=[0.5 0.5 0.5 1.0]  GraphicAmbientColor=[0.15 0.15 0.15 1.0]  GraphicEmissiveColor=[0.0 0.0 0.0 1.0]  GraphicShininess=75  DoExposeReferenceFrame=off  SerializedFrames=<Frames><Frame><Id>Frame1</Id><Value><Name>MainFrameRev</Name><Origin><Source>GeometricFeature</Source><FeatureName>circular curve 11</FeatureName></Origin><PrimaryAxis><DefinedDirection>-Z</DefinedDirection><Source>GeometricFeature</Source><SourceDirection>+Z</SourceDirection><FeatureName>segment 13</FeatureName></PrimaryAxis><SecondaryAxis><DefinedDirection>+X</DefinedDirection><Source>ReferenceFrame</Source><SourceDirection>+X</SourceDirection><FeatureName></FeatureName></SecondaryAxis></Value></Frame><Frame><Id>Frame2</Id><Value><Name>ArticulationCyl</Name><Origin><Source>GeometricFeature</Source><FeatureName>circular curve 5</FeatureName></Origin><PrimaryAxis><DefinedDirection>-Z</DefinedDirection><Source>GeometricFeature</Source><SourceDirection>+Z</SourceDirection><FeatureName>segment 7</FeatureName></PrimaryAxis><SecondaryAxis><DefinedDirection>+X</DefinedDirection><Source>ReferenceFrame</Source><SourceDirection>+X</SourceDirection><FeatureName></FeatureName></SecondaryAxis></Value></Frame></Frames>
  ArticulationRodSolid : sm_lib/Body Elements/File Solid  ExtGeomFileName=ArticulationPiston.step  UnitType=FromFile  ExtGeomFileUnits=m  StepReaderType=HEX  ExportConvexHullGeometry=off  InertiaType=CalculateFromGeometry  BasedOnType=Mass  Density=1000  DensityUnits=kg/m^3  Mass=motGradParams.articulation.rod.mass  MassUnits=kg  CenterOfMass=[0 0 0]  CenterOfMassUnits=m  MomentsOfInertia=[1 1 1]  MomentsOfInertiaUnits=kg*m^2  ProductsOfInertia=[0 0 0]  ProductsOfInertiaUnits=kg*m^2  GraphicType=FromGeometry  MarkerShape=Sphere  MarkerSize=10  GraphicVisPropType=SimpleVisualProperties  GraphicDiffuseColor=mtrgrd.clr.artic_rod  GraphicOpacity=1  GraphicSpecularColor=[0.5 0.5 0.5 1.0]  GraphicAmbientColor=[0.15 0.15 0.15 1.0]  GraphicEmissiveColor=[0.0 0.0 0.0 1.0]  GraphicShininess=75  DoExposeReferenceFrame=off  SerializedFrames=<Frames><Frame><Id>Frame1</Id><Value><Name>RearFrame</Name><Origin><Source>GeometricFeature</Source><FeatureName>circular curve 4</FeatureName></Origin><PrimaryAxis><DefinedDirection>+Z</DefinedDirection><Source>ReferenceFrame</Source><SourceDirection>+Z</SourceDirection><FeatureName></FeatureName></PrimaryAxis><SecondaryAxis><DefinedDirection>+X</DefinedDirection><Source>ReferenceFrame</Source><SourceDirection>+X</SourceDirection><FeatureName></FeatureName></SecondaryAxis></Value></Frame><Frame><Id>Frame2</Id><Value><Name>ArticulationCyl</Name><Origin><Source>GeometricFeature</Source><FeatureName>planar surface 1</FeatureName></Origin><PrimaryAxis><DefinedDirection>-Z</DefinedDirection><Source>GeometricFeature</Source><SourceDirection>+Z</SourceDirection><FeatureName>segment 10</FeatureName></PrimaryAxis><SecondaryAxis><DefinedDirection>+X</DefinedDirection><Source>ReferenceFrame</Source><SourceDirection>+X</SourceDirection><FeatureName></FeatureName></SecondaryAxis></Value></Frame></Frames>
  Cylindrical Rod : sm_lib/Joints/Cylindrical Joint  JointMode=Normal  CompositeWrenchDir=FollowerOnBase  CompositeWrenchFrame=BaseFrame  SenseConstraintForce=off  SenseConstraintTorque=off  SenseTotalForce=off  SenseTotalTorque=off  RzPositionTargetSpecify=off  RzPositionTargetPriority=High  RzPositionTargetValue=0  RzPositionTargetValueUnits=deg  RzVelocityTargetSpecify=off  RzVelocityTargetPriority=High  RzVelocityTargetValue=0  RzVelocityTargetValueUnits=deg/s  RzEquilibriumPosition=0  RzEquilibriumPositionUnits=deg  RzSpringStiffness=0  RzSpringStiffnessUnits=N*m/deg  RzDampingCoefficient=0  RzDampingCoefficientUnits=N*m/(deg/s)  RzLowerLimitSpecify=off  RzLowerLimitBound=-90  RzLowerLimitBoundUnits=deg  RzLowerLimitStiffness=1e4  RzLowerLimitStiffnessUnits=N*m/deg  RzLowerLimitDamping=10  RzLowerLimitDampingUnits=N*m/(deg/s)  RzLowerLimitTransitionRegionWidth=0.1  RzLowerLimitTransitionRegionWidthUnits=deg  RzUpperLimitSpecify=off  RzUpperLimitBound=90  RzUpperLimitBoundUnits=deg  RzUpperLimitStiffness=1e4  RzUpperLimitStiffnessUnits=N*m/deg  RzUpperLimitDamping=10  RzUpperLimitDampingUnits=N*m/(deg/s)  RzUpperLimitTransitionRegionWidth=0.1  RzUpperLimitTransitionRegionWidthUnits=deg  RzTorqueActuationMode=NoTorque  RzMotionActuationMode=ComputedMotion  RzSensePosition=off  RzSenseVelocity=off  RzSenseAcceleration=off  RzSenseTorqueForce=off  RzSenseLowerLimitTorqueForce=off  RzSenseUpperLimitTorqueForce=off  PzPositionTargetSpecify=off  PzPositionTargetPriority=High  PzPositionTargetValue=0  PzPositionTargetValueUnits=m  PzVelocityTargetSpecify=off  PzVelocityTargetPriority=High  PzVelocityTargetValue=0  PzVelocityTargetValueUnits=m/s  PzEquilibriumPosition=0  PzEquilibriumPositionUnits=m  PzSpringStiffness=0  PzSpringStiffnessUnits=N/m  PzDampingCoefficient=0  PzDampingCoefficientUnits=N/(m/s)  PzLowerLimitSpecify=off  PzLowerLimitBound=-1  PzLowerLimitBoundUnits=m  PzLowerLimitStiffness=1e6  PzLowerLimitStiffnessUnits=N/m  PzLowerLimitDamping=1e3  PzLowerLimitDampingUnits=N/(m/s)  PzLowerLimitTransitionRegionWidth=1e-4  PzLowerLimitTransitionRegionWidthUnits=m  PzUpperLimitSpecify=off  PzUpperLimitBound=1  PzUpperLimitBoundUnits=m  PzUpperLimitStiffness=1e6  PzUpperLimitStiffnessUnits=N/m  PzUpperLimitDamping=1e3  PzUpperLimitDampingUnits=N/(m/s)  PzUpperLimitTransitionRegionWidth=1e-4  PzUpperLimitTransitionRegionWidthUnits=m  PzTorqueActuationMode=NoTorque  PzMotionActuationMode=ComputedMotion  PzSensePosition=off  PzSenseVelocity=off  PzSenseAcceleration=off  PzSenseTorqueForce=off  PzSenseLowerLimitTorqueForce=off  PzSenseUpperLimitTorqueForce=off
  Revolute Cyl : sm_lib/Joints/Revolute Joint  JointMode=Normal  CompositeWrenchDir=FollowerOnBase  CompositeWrenchFrame=BaseFrame  SenseConstraintForce=off  SenseConstraintTorque=off  SenseTotalForce=off  SenseTotalTorque=off  PositionTargetSpecify=off  PositionTargetPriority=High  PositionTargetValue=0  PositionTargetValueUnits=deg  VelocityTargetSpecify=off  VelocityTargetPriority=High  VelocityTargetValue=0  VelocityTargetValueUnits=deg/s  EquilibriumPosition=0  EquilibriumPositionUnits=deg  SpringStiffness=0  SpringStiffnessUnits=N*m/deg  DampingCoefficient=0  DampingCoefficientUnits=N*m/(deg/s)  LowerLimitSpecify=off  LowerLimitBound=-90  LowerLimitBoundUnits=deg  LowerLimitStiffness=1e4  LowerLimitStiffnessUnits=N*m/deg  LowerLimitDamping=10  LowerLimitDampingUnits=N*m/(deg/s)  LowerLimitTransitionRegionWidth=0.1  LowerLimitTransitionRegionWidthUnits=deg  UpperLimitSpecify=off  UpperLimitBound=90  UpperLimitBoundUnits=deg  UpperLimitStiffness=1e4  UpperLimitStiffnessUnits=N*m/deg  UpperLimitDamping=10  UpperLimitDampingUnits=N*m/(deg/s)  UpperLimitTransitionRegionWidth=0.1  UpperLimitTransitionRegionWidthUnits=deg  TorqueActuationMode=NoTorque  MotionActuationMode=ComputedMotion  SensePosition=off  SenseVelocity=off  SenseAcceleration=off  SenseTorqueForce=off  SenseLowerLimitTorqueForce=off  SenseUpperLimitTorqueForce=off
  R : PMIOPort  Side=Left
  F : PMIOPort  Port=2  Side=Left
  B : PMIOPort  Port=3  Side=Right
  m : Outport
  wires:
  In Bus Element/1 -> Actuator/1(p)
  Actuator/1(m) -> m/1
  connections:
  Revolute Cyl/RConn1 -- ArticulationCylSolid/LConn1
  Revolute Cyl/LConn1 -- B/RConn1
  Cylindrical Rod/LConn1 -- F/RConn1
  Cylindrical Rod/RConn1 -- ArticulationRodSolid/LConn1
  Actuator/LConn1 -- R/RConn1
  Actuator/LConn2 -- ArticulationCylSolid/RConn1
  Actuator/RConn1 -- ArticulationRodSolid/RConn1

== system sm_motor_grader_Drive_Steer/Config ==
  Mechanism Configuration : sm_lib/Utilities/Mechanism Configuration  UniformGravity=Constant  GravityVector=[0 0 -9.80665]  GravityVectorUnits=m/s^2  LinearizationDelta=0.001  JointModeTransitionNonlinearIterations=2
  Solver Configuration : nesl_utility/Solver Configuration  PhysicalDomain=network_engine_domain  SubClassName=solver  LeftPortType=input  RightPortType=generic  Tones=[]  Harmonics=[]  SimulateNoise=off  Profile=off  UseLocalSampling=off  EnableSwitchedLinearOptims=on  FrequencyDomain=off  UseCCode=off  RelTol=0.001  AbsTol=1e-06  MinStep=1e-09  ToWorkspace=off  RevertToSquareIcSolve=off  NumHomotopyIterations=100  PhasorMode=off  PhasorModeNumHarmonics=1  ConsistencySolver=NEWTON_XTOL_AFTER_FTOL  IndexReductionMethod=DerivativeReplacement  DoDC=off  ResidualTolerance=1e-09  ConsistencyTolSource=GLOBAL  ConsistencyAbsTol=0.001  ConsistencyRelTol=0.001  ConsistencyTolFactor=0.001  UseLocalSolver=off  LocalSolverChoice=NE_BACKWARD_EULER_ADVANCER  ResolveIndetEquations=on  FunctionEvalNumThread=1  LocalSolverSampleTime=0.001  DoFixedCost=off  MaxNonlinIter=3  MaxModeIter=2  ComputeImpulses=off  ImpulseIterations=2  LinearAlgebra=Sparse  LinearAlgebraNumThread=0  EquationFormulation=NE_TIME_EF  DelaysMemoryBudget=1024  AutomaticFiltering=on  FilteringTimeConstant=0.001  PartitionStorageMethod=AS_NEEDED  PartitionMemoryBudget=1024  PartitionMethod=FAST  MultibodyUseLocalSolver=off  MultibodyLocalSolverChoice=ODE1  MultibodyLocalSolverSampleTime=0.001
  W : PMIOPort  Side=Left
  connections:
  Mechanism Configuration/RConn1 -- W/RConn1 -- Solver Configuration/RConn1

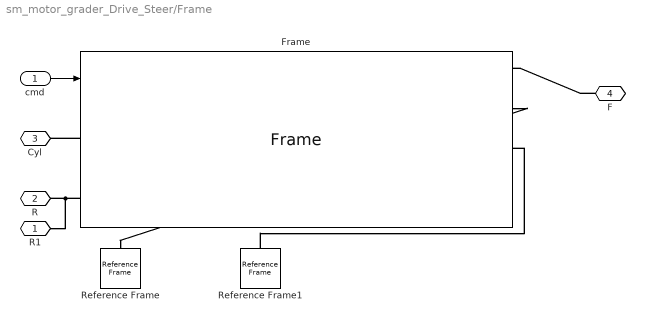
== system sm_motor_grader_Drive_Steer/Frame ==
  cmd : Inport
  Frame : sm_motor_grader_lib/Frame
  Reference Frame : sm_lib/Frames and Transforms/Reference Frame
  Reference Frame1 : sm_lib/Frames and Transforms/Reference Frame
  R1 : PMIOPort  Side=Right
  R : PMIOPort  Port=2  Side=Right
  Cyl : PMIOPort  Port=3  Side=Right
  F : PMIOPort  Port=4  Side=Right
  wires:
  cmd/1 -> Frame/1
  connections:
  Frame/LConn1 -- Cyl/RConn1
  R1/RConn1 -- Frame/LConn2 -- R/RConn1
  Frame/RConn3 -- Reference Frame/RConn1
  Reference Frame1/RConn1 -- Frame/RConn5
  F/RConn1 -- Frame/RConn1

== system sm_motor_grader_Drive_Steer/Inputs ==
  m : Inport
  Control : sm_motor_grader_lib/Control  SystemSampleTime=-1  VariantControl=Control  VariantActivationTime=update diagram  AllowFlexibleInterface=on  Latency=0  AutoFrameSizeCalculation=off
  Data : sm_motor_grader_lib/Data  SystemSampleTime=-1  VariantControl=Data  VariantActivationTime=update diagram  AllowFlexibleInterface=on  Latency=0  AutoFrameSizeCalculation=off
  Test : Outport

== system sm_motor_grader_Drive_Steer/Motor Grader ==
  Vehicle : Subsystem
  F : PMIOPort  Side=Right
  connections:
  Vehicle/RConn1 -- F/RConn1

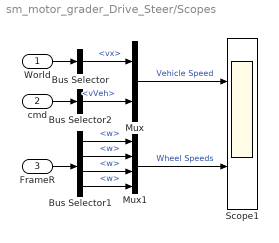
== system sm_motor_grader_Drive_Steer/Scopes ==
  World : Inport
  cmd : Inport  Port=2
  FrameR : Inport  Port=3
  Bus Selector : BusSelector  OutputSignals=vx
  Bus Selector1 : BusSelector  OutputSignals=WhlFL.w,WhlFR.w,WhlRL.w,WhlRR.w
  Bus Selector2 : BusSelector  OutputSignals=vVeh
  Mux : Mux  Inputs=2
  Mux1 : Mux
  Scope1 : Scope  NumInputPorts=2
  wires:
  Bus Selector1/4 -> Mux1/4  "<w>"
  cmd/1 -> Bus Selector2/1
  Bus Selector1/2 -> Mux1/2  "<w>"
  Bus Selector/1 -> Mux/1  "<vx>"
  Bus Selector2/1 -> Mux/2  "<vVeh>"
  Bus Selector1/1 -> Mux1/1  "<w>"
  Bus Selector1/3 -> Mux1/3  "<w>"
  FrameR/1 -> Bus Selector1/1
  Mux1/1 -> Scope1/2  "Wheel Speeds"
  World/1 -> Bus Selector/1
  Mux/1 -> Scope1/1  "Vehicle Speed"

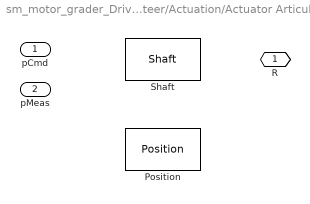
== system sm_motor_grader_Drive_Steer/Actuation/Actuator Articulation ==
  pCmd : Inport
  pMeas : Inport  Port=2
  Position : sm_motor_grader_lib/Position  VariantControl=Position
  Shaft : sm_motor_grader_lib/Shaft  VariantControl=Shaft  Kp=motGradParams.articulation.propGain  Ki=motGradParams.articulation.integral  Kd=motGradParams.articulation.derivative  p_init=motGradParams.articulation.initPos
  R : PMIOPort  Side=Right

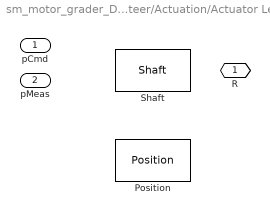
== system sm_motor_grader_Drive_Steer/Actuation/Actuator LeanL ==
  pCmd : Inport
  pMeas : Inport  Port=2
  Position : sm_motor_grader_lib/Position  VariantControl=Position
  Shaft : sm_motor_grader_lib/Shaft  VariantControl=Shaft  Kp=motGradParams.wheelLean.propGain  Ki=motGradParams.wheelLean.integral  Kd=motGradParams.wheelLean.derivative  p_init=motGradParams.wheelLean.initPos
  R : PMIOPort  Side=Right

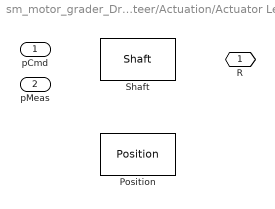
== system sm_motor_grader_Drive_Steer/Actuation/Actuator LeanR ==
  pCmd : Inport
  pMeas : Inport  Port=2
  Position : sm_motor_grader_lib/Position  VariantControl=Position
  Shaft : sm_motor_grader_lib/Shaft  VariantControl=Shaft  Kp=motGradParams.wheelLean.propGain  Ki=motGradParams.wheelLean.integral  Kd=motGradParams.wheelLean.derivative  p_init=motGradParams.wheelLean.initPos
  R : PMIOPort  Side=Right

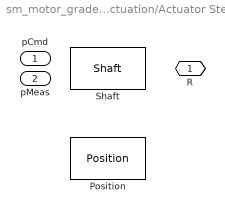
== system sm_motor_grader_Drive_Steer/Actuation/Actuator SteerL ==
  pCmd : Inport
  pMeas : Inport  Port=2
  Position : sm_motor_grader_lib/Position  VariantControl=Position
  Shaft : sm_motor_grader_lib/Shaft  VariantControl=Shaft  Kp=motGradParams.steer.propGain  Ki=motGradParams.steer.integral  Kd=motGradParams.steer.derivative  p_init=motGradParams.steer.initPos
  R : PMIOPort  Side=Right

== system sm_motor_grader_Drive_Steer/Actuation/Actuator SteerR ==
  pCmd : Inport
  pMeas : Inport  Port=2
  Position : sm_motor_grader_lib/Position  VariantControl=Position
  Shaft : sm_motor_grader_lib/Shaft  VariantControl=Shaft  Kp=motGradParams.steer.propGain  Ki=motGradParams.steer.integral  Kd=motGradParams.steer.derivative  p_init=motGradParams.steer.initPos
  R : PMIOPort  Side=Right

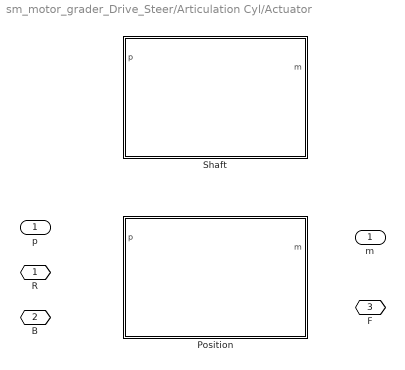
== system sm_motor_grader_Drive_Steer/Articulation Cyl/Actuator ==
  p : Inport
  Position : Subsystem  VariantControl=Position
      mask Display: image('sm_motor_grader_cyljoint_Position_IMAGE.png')
  Shaft : Subsystem  VariantControl=Shaft
      mask Display: image('sm_motor_grader_cyljoint_Shaft_IMAGE.png')
  R : PMIOPort  Side=Left
  B : PMIOPort  Port=2  Side=Left
  F : PMIOPort  Port=3  Side=Right
  m : Outport

== system sm_motor_grader_Drive_Steer/Motor Grader/Vehicle ==
  Camera Frames : sm_vehicle_utilities_lib/Camera Frames  Camera=Camera  popup_dolly_camera=Off
  F : PMIOPort  Side=Right
  connections:
  Camera Frames/RConn1 -- F/RConn1
